simulink model "pi_p_controller"  (R2018a)
settings: Solver=VariableStepAuto  StartTime=0.0  StopTime=1  RelTol=1e-3
undefined symbols (not defined in the file or in its folder): p
libraries: cstblocks x2
settings Model: Creator=mz-171742  LastModifiedBy=mz-171742

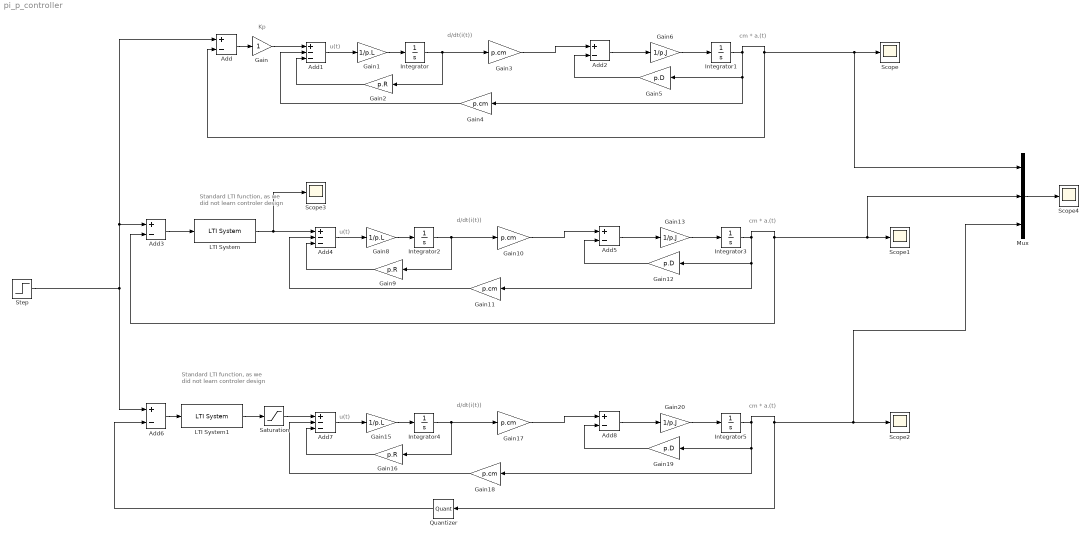
== system pi_p_controller ==
  note: Standard LTI function,
      | as we did not learn
      | controler design
  note: d/dt(i(t))
  note: cm * a.(t)
  note: u(t)
  note: Kp
  note: u(t)
  note: cm * a.(t)
  note: d/dt(i(t))
  note: u(t)
  note: cm * a.(t)
  note: d/dt(i(t))
  note: Standard LTI function,
      | as we did not learn
      | controler design
  Add{,2..3,5..6,8} (6 alike) : Sum  Inputs=+-
  Add1 : Sum  Inputs=+--
  Add4 : Sum  Inputs=+--
  Add7 : Sum  Inputs=+--
  Gain : Gain
  Gain1 : Gain  Gain=1/p.L
  Gain{3..4,10..11,17..18} (6 alike) : Gain  Gain=p.cm
  Gain12 : Gain  Gain=p.D
  Gain13 : Gain  Gain=1/p.J
  Gain15 : Gain  Gain=1/p.L
  Gain16 : Gain  Gain=p.R
  Gain19 : Gain  Gain=p.D
  Gain2 : Gain  Gain=p.R
  Gain20 : Gain  Gain=1/p.J
  Gain5 : Gain  Gain=p.D
  Gain6 : Gain  Gain=1/p.J
  Gain8 : Gain  Gain=1/p.L
  Gain9 : Gain  Gain=p.R
  Integrator{,1..5} (6 alike) : Integrator
  LTI System : cstblocks/LTI System  sys=tf(1,[1 1])  IC=[]
  LTI System1 : cstblocks/LTI System  sys=tf(1,[1 1])  IC=[]
  Mux : Mux  Inputs=3
  Quantizer : Quantizer
  Saturation : Saturate
  Scope{,1..4} (5 alike) : Scope
  Step : Step  Time=0  SampleTime=0
  wires:
  Gain2/1 -> Add1/3
  Gain4/1 -> Add1/2
  Add2/1 -> Gain6/1
  Gain6/1 -> Integrator1/1
  Add/1 -> Gain/1
  Gain1/1 -> Integrator/1
  Gain3/1 -> Add2/1
  Gain/1 -> Add1/1
  Integrator1/1 -> Add/2, Mux/1, Scope/1, Gain4/1, Gain5/1
  Integrator/1 -> Gain2/1, Gain3/1
  Add1/1 -> Gain1/1
  Gain5/1 -> Add2/2
  Gain8/1 -> Integrator2/1
  Gain10/1 -> Add5/1
  Add5/1 -> Gain13/1
  Gain13/1 -> Integrator3/1
  Gain11/1 -> Add4/2
  Add4/1 -> Gain8/1
  Integrator2/1 -> Gain9/1, Gain10/1
  Gain9/1 -> Add4/3
  Integrator3/1 -> Add3/2, Mux/2, Scope1/1, Gain11/1, Gain12/1
  Gain12/1 -> Add5/2
  Gain15/1 -> Integrator4/1
  Gain17/1 -> Add8/1
  Add8/1 -> Gain20/1
  Gain20/1 -> Integrator5/1
  Gain18/1 -> Add7/2
  Add7/1 -> Gain15/1
  Step/1 -> Add6/1, Add3/1, Add/1
  Integrator4/1 -> Gain16/1, Gain17/1
  Gain16/1 -> Add7/3
  Integrator5/1 -> Quantizer/1, Mux/3, Scope2/1, Gain18/1, Gain19/1
  Gain19/1 -> Add8/2
  Add3/1 -> LTI System/1
  LTI System/1 -> Add4/1, Scope3/1
  Add6/1 -> LTI System1/1
  LTI System1/1 -> Saturation/1
  Saturation/1 -> Add7/1
  Quantizer/1 -> Add6/2
  Mux/1 -> Scope4/1
